simulink model "Pacemaker"  (R2020a)
settings: Solver=FixedStepAuto  StartTime=0.0  StopTime=10.0  FixedStep=1e-3  RelTol=1e-3  EnableMultiTasking=on
undefined symbols (not defined in the file or in its folder): A1, D0, D1, D10, D11, D12, D2, D3, D4, D5, D6, D7, D8, D9, PTA0, PTA1, PTA2, PTB23, PTB3, PTB9, PTC16, PTC17, PTC2, PTC3, PTC4, PTD0, PTD2, PTD3
libraries: frdmk64flib x16
settings Model: ExtModeTrigDuration=5  Creator=John Sarga  LastModifiedBy=John Sarga
settings OptimizationCC: EnhancedBackFolding=on  PassReuseOutputArgsAs=Individual arguments  ZeroExternalMemoryAtStartup=off  ZeroInternalMemoryAtStartup=off  MaxStackSize=64  OptimizeBlockOrder=speed  DifferentSizesBufferReuse=on  OptimizationCustomize=off  EfficientTunableParamExpr=on
settings DebuggingCC: ParameterTunabilityLossMsg=error
settings HardwareCC: ProdBitPerPointer=32  ProdBitPerSizeT=32  ProdBitPerPtrDiffT=32  ProdLargestAtomicInteger=Long  ProdLargestAtomicFloat=Double  ProdWordSize=32  ProdHWDeviceType=ARM Compatible->ARM Cortex
settings SFSimCC: MATLABDynamicMemAlloc=off
settings RTWCC: SystemTargetFile=ert.tlc  HardwareBoard=NXP FRDM-K64F  TemplateMakefile=ert_default_tmf  Toolchain=GNU Tools for ARM Embedded Processors
settings CodeAppCC: ForceParamTrailComments=on  IgnoreCustomStorageClasses=off  OperatorAnnotations=on  SimulinkDataObjDesc=on  SFDataObjDesc=on  InsertBlockDesc=on

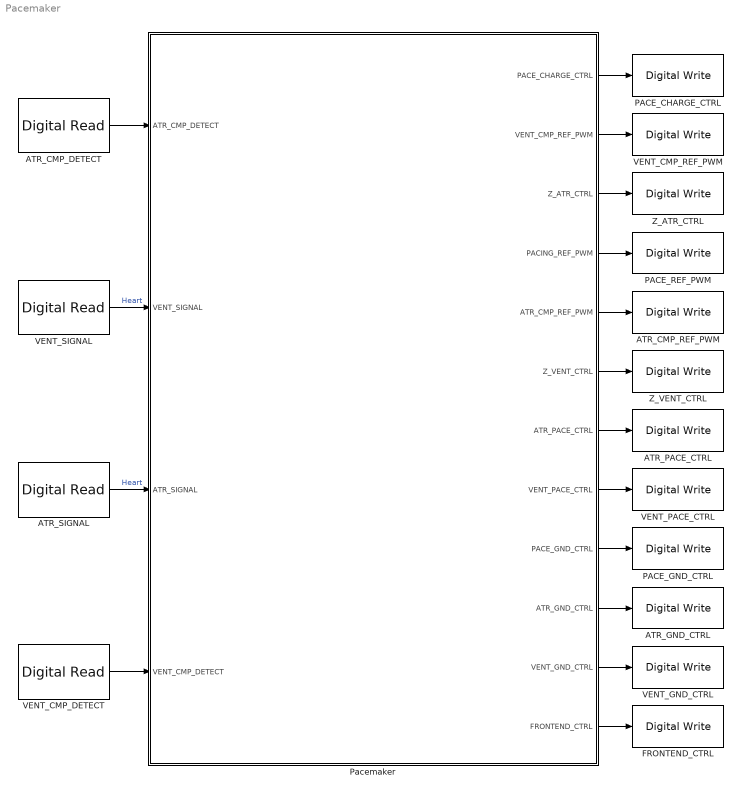
== system Pacemaker ==
  ATR_CMP_DETECT : frdmk64flib/Digital Read  Whichpin=PTC16 (D0)  SampleTime=-1
  ATR_CMP_REF_PWM : frdmk64flib/Digital Write  Whichpin=PTC2 (D6)
  ATR_GND_CTRL : frdmk64flib/Digital Write  Whichpin=PTD2 (D11)
  ATR_PACE_CTRL : frdmk64flib/Digital Write  Whichpin=PTA0 (D8)
  ATR_SIGNAL : frdmk64flib/Digital Read  Whichpin=PTB3 (A1)  SampleTime=-1
  FRONTEND_CTRL : frdmk64flib/Digital Write  Whichpin=PTD3 (D12)
  PACE_CHARGE_CTRL : frdmk64flib/Digital Write  Whichpin=PTB9 (D2)
  PACE_GND_CTRL : frdmk64flib/Digital Write  Whichpin=PTD0 (D10)
  PACE_REF_PWM : frdmk64flib/Digital Write  Whichpin=PTA2 (D5)
  Pacemaker : Stateflow chart  TreatAsAtomicUnit=on
      settings: PortSchema="{\"entries\":[{\"content\":{\"sides\":[{\"content\":{\"connectorIds\":[\"In1\",\"In2\",\"In3\",\"In4\"]},\"type\":\"ConnectorPlacement.EquallySpacedRectSide\",\"uuid\":\"65eaab6b-31c5-41c7-a958-8496cb1dd2e8\"},{\"content\":{\"connectorIds\":[\"Out4\",\"Out2\",\"Out8\",\"Out6\",\"Out5\",\"Out9\",\"Out1\",\"Out3\",\"Out7\",\"Out10\",\"Out11\",\"Out12\"],\"side\":\"RIGHT\"},\"type\":\"ConnectorPlacement.EquallySpacedRectSide\",\"uuid\":\"e3fe0d49-d364-480e-9c1d-e672590667d9\"},{\"content\":{\"connectorIds\":[],\"side\":\"TOP\"},\"type\":\"ConnectorPlacement.EquallySpacedRectSide\",\"uuid\":\"d1dc7c5b-2428-4c6e-96f9-9594e2e7aeeb\"}]},\"type\":\"ConnectorPlacement.EquallySpacedConnector\",\"uuid\":\"50016c44-f69e-4f27-b5a8-fdf179f0e08a\"}],\"packageUris\":[\"http://schema.mathworks.com/mf0/Connector/19700101\"],\"version\":\"1.0\"}"
  VENT_CMP_DETECT : frdmk64flib/Digital Read  Whichpin=PTC17 (D1)  SampleTime=-1
  VENT_CMP_REF_PWM : frdmk64flib/Digital Write  Whichpin=PTA1 (D3)
  VENT_GND_CTRL : frdmk64flib/Digital Write  Whichpin=PTD3 (D12)
  VENT_PACE_CTRL : frdmk64flib/Digital Write  Whichpin=PTC4 (D9)
  VENT_SIGNAL : frdmk64flib/Digital Read  Whichpin=PTB3 (A1)  SampleTime=-1
  Z_ATR_CTRL : frdmk64flib/Digital Write  Whichpin=PTB23 (D4)
  Z_VENT_CTRL : frdmk64flib/Digital Write  Whichpin=PTC3 (D7)
  wires:
  Pacemaker/12(FRONTEND_CTRL) -> FRONTEND_CTRL/1
  Pacemaker/7(PACE_GND_CTRL) -> PACE_GND_CTRL/1
  Pacemaker/5(ATR_CMP_REF_PWM) -> ATR_CMP_REF_PWM/1
  ATR_CMP_DETECT/1 -> Pacemaker/1(ATR_CMP_DETECT)
  VENT_CMP_DETECT/1 -> Pacemaker/4(VENT_CMP_DETECT)
  Pacemaker/3(VENT_PACE_CTRL) -> VENT_PACE_CTRL/1
  Pacemaker/4(PACE_CHARGE_CTRL) -> PACE_CHARGE_CTRL/1
  Pacemaker/9(Z_VENT_CTRL) -> Z_VENT_CTRL/1
  Pacemaker/6(PACING_REF_PWM) -> PACE_REF_PWM/1
  Pacemaker/8(Z_ATR_CTRL) -> Z_ATR_CTRL/1
  Pacemaker/2(VENT_CMP_REF_PWM) -> VENT_CMP_REF_PWM/1
  Pacemaker/10(ATR_GND_CTRL) -> ATR_GND_CTRL/1
  VENT_SIGNAL/1 -> Pacemaker/2(VENT_SIGNAL)  "Heart"
  Pacemaker/11(VENT_GND_CTRL) -> VENT_GND_CTRL/1
  Pacemaker/1(ATR_PACE_CTRL) -> ATR_PACE_CTRL/1
  ATR_SIGNAL/1 -> Pacemaker/3(ATR_SIGNAL)  "Heart"

== stateflow chart Pacemaker/Pacemaker ==
  state Off
    p_pacingMode = Off
    ATR_PACE_CTRL = 0
  state AOO
    state Charging
      ATR_PACE_CTRL = 0
      VENT_PACE_CTRL = 0
      PACE_CHARGE_CTRL = 1
      PACING_REF_PWM = 0.3
    state Discharging
      PACE_CHARGE_CTRL = 0
      PACE_GND_CTRL  = 1
      ATR_PACE_CTRL = 0
      VENT_PACE_CTRL = 0
      Z_ATR_CTRL = 0
      Z_VENT_CTRL = 0
    (default) -> Charging
  (default) -> Off : {p_pacingMode = 0;}
  AOO -> Off : [p_pacingMode == Off]
  Off -> AOO : [p_pacingMode == AOO]
  data: ATR_PACE_CTRL output boolean; VENT_CMP_REF_PWM output; p_pacingMode local Enum: PacemakerMode; VENT_PACE_CTRL output boolean; PACE_CHARGE_CTRL output; ATR_CMP_REF_PWM output; PACING_REF_PWM output boolean; PACE_GND_CTRL output boolean; Z_ATR_CTRL output boolean; Z_VENT_CTRL output boolean; ATR_CMP_DETECT input boolean; VENT_SIGNAL input boolean; ATR_SIGNAL input boolean; VENT_CMP_DETECT input boolean; ATR_GND_CTRL output boolean; VENT_GND_CTRL output boolean; FRONTEND_CTRL output boolean
